simulink model "Simulink Library"  (R2018b)
settings: Solver=FixedStepAuto  StartTime=0.0  StopTime=10.0  RelTol=1e-3
undefined symbols (not defined in the file or in its folder): Battery, GYRO, LME, LRLI, MODE, MSE, PING, RME, RRLI
libraries: legoev3lib x36, simulink x33, dspstat3 x5, dspmtrx3 x3, fuzblock x2, simulink_extras x1
(part 2 of 2)

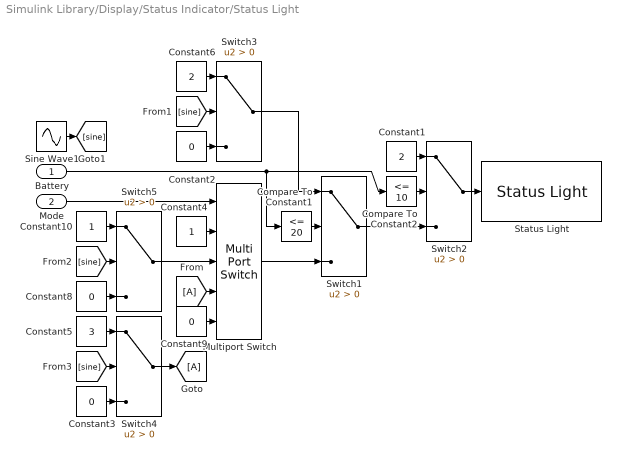
== system Simulink Library/Display/Status Indicator/Status Light ==
  Battery : Inport
  Mode : Inport  Port=2
  Compare To Constant1 : simulink/Logic and Bit Operations/Compare To Constant  relop=<=  const=20  OutDataTypeStr=boolean
  Compare To Constant2 : simulink/Logic and Bit Operations/Compare To Constant  relop=<=  const=10  OutDataTypeStr=boolean
  Constant1 : Constant  Value=2
  Constant10 : Constant
  Constant{2..3,8..9} (4 alike) : Constant  Value=0
  Constant4 : Constant
  Constant5 : Constant  Value=3
  Constant6 : Constant  Value=2
  Multiport Switch : MultiPortSwitch  DataPortOrder=Zero-based contiguous  Inputs=4  DiagnosticForDefault=None  zeroidx=on
  Sine Wave1 : Sin  SineType=Sample based  Samples=100  SampleTime=0.01
  Status Light : legoev3lib/Status Light
      settings: SourceProductName=Simulink Support Package for LEGO MINDSTORMS EV3 Hardware  SourceProductBaseCode=LEGOEV3
  Switch{1..5} (5 alike) : Switch  Criteria=u2 > Threshold
  wires:
  Multiport Switch/1 -> Switch1/3
  Compare To Constant2/1 -> Switch2/2
  Switch2/1 -> Status Light/1
  Battery/1 -> Compare To Constant2/1, Compare To Constant1/1
  Compare To Constant1/1 -> Switch1/2
  Switch1/1 -> Switch2/3
  Switch3/1 -> Switch1/1
  Mode/1 -> Multiport Switch/1
  Constant4/1 -> Multiport Switch/2
  Switch5/1 -> Multiport Switch/3
  [A] -> Multiport Switch/4
  Constant9/1 -> Multiport Switch/5
  [sine] -> Switch3/2
  Constant6/1 -> Switch3/1
  Constant2/1 -> Switch3/3
  Constant1/1 -> Switch2/1
  Constant5/1 -> Switch4/1
  [sine] -> Switch4/2
  Constant3/1 -> Switch4/3
  Constant10/1 -> Switch5/1
  [sine] -> Switch5/2
  Constant8/1 -> Switch5/3
  Switch4/1 -> [A]
  Sine Wave1/1 -> [sine]

== system Simulink Library/Motor Logic/Trim Logic/Trim High Spd ==
  Trim In : Inport
  Add2 : Sum  Inputs=+-
  Compare To Constant1 : simulink/Logic and Bit Operations/Compare To Constant  relop=>  const=0  OutDataTypeStr=boolean
  Compare To Constant2 : simulink/Logic and Bit Operations/Compare To Constant  relop=<  const=0  OutDataTypeStr=boolean
  Constant3 : Constant  Value=10
  Gain : Gain  Gain=-1
  Gain1 : Gain  Gain=-1
  Switch1 : Switch  Criteria=u2 > Threshold
  Switch2 : Switch  Criteria=u2 > Threshold
  Trim Right : Outport
  Trim Left : Outport  Port=2
  wires:
  Trim In/1 -> Add2/1
  Constant3/1 -> Add2/2
  Add2/1 -> Compare To Constant2/1, Switch2/1, Switch1/1, Compare To Constant1/1
  Compare To Constant1/1 -> Switch1/3, Switch1/2
  Compare To Constant2/1 -> Switch2/3, Switch2/2
  Switch1/1 -> Gain/1
  Gain/1 -> Trim Right/1
  Switch2/1 -> Gain1/1
  Gain1/1 -> Trim Left/1

== system Simulink Library/Motor Logic/Trim Logic/Trim Low Spd ==
  Trim In : Inport
  Add2 : Sum  Inputs=+-
  Compare To Constant1 : simulink/Logic and Bit Operations/Compare To Constant  relop=>  const=0  OutDataTypeStr=boolean
  Compare To Constant2 : simulink/Logic and Bit Operations/Compare To Constant  relop=<  const=0  OutDataTypeStr=boolean
  Constant3 : Constant  Value=10
  Switch1 : Switch  Criteria=u2 > Threshold
  Switch2 : Switch  Criteria=u2 > Threshold
  Trim Right : Outport
  Trim Left : Outport  Port=2
  wires:
  Trim In/1 -> Add2/1
  Constant3/1 -> Add2/2
  Add2/1 -> Compare To Constant2/1, Switch2/1, Switch1/1, Compare To Constant1/1
  Compare To Constant1/1 -> Switch1/3, Switch1/2
  Compare To Constant2/1 -> Switch2/3, Switch2/2
  Switch1/1 -> Trim Right/1
  Switch2/1 -> Trim Left/1

== system Simulink Library/PathTracking/Control Logic/Battery Bias ==
  Batt_Lvl : Inport
  Ceil : Rounding
  Constant : Constant
  Direct Lookup Table (n-D) : LookupNDDirect  NumberOfTableDimensions=1  Table=[0.256 0.128 0.064 0.032 0.016 0.008 0.004 0.002 0.001 0];
  Gain : Gain  Gain=0.1
  Sum : Sum  Inputs=|++
  Battery Bias : Outport
  wires:
  Direct Lookup Table (n-D)/1 -> Sum/1
  Constant/1 -> Sum/2
  Sum/1 -> Battery Bias/1
  Gain/1 -> Ceil/1
  Ceil/1 -> Direct Lookup Table (n-D)/1
  Batt_Lvl/1 -> Gain/1

== system Simulink Library/PathTracking/Control Logic/LP Filter && d//dt ==
  LightError : Inport
  Gain : Gain  Gain=1/0.01
  Low Pass Filter : DiscreteFilter  Numerator=[.2]  Denominator=[1 -0.8]
  Sum3 : Sum  Inputs=+-
  Unit Delay : UnitDelay  SampleTime=-1
  LightErrorDot : Outport
  wires:
  Unit Delay/1 -> Sum3/2
  Gain/1 -> Unit Delay/1, Sum3/1
  Sum3/1 -> LightErrorDot/1  "theta_dot"
  Low Pass Filter/1 -> Gain/1
  LightError/1 -> Low Pass Filter/1

== system Simulink Library/PathTracking/Control Logic/PID Bias ==
  RLI Error : Inport
  Abs : Abs
  Constant : Constant  Value=4
  Constant1 : Constant  Value=-4
  Switch1 : Switch  Criteria=u2 > Threshold  Threshold=30
  Switch2 : Switch  Criteria=u2 > Threshold
  PID_Bias : Outport
  wires:
  Switch1/1 -> PID_Bias/1
  RLI Error/1 -> Switch2/2, Abs/1
  Abs/1 -> Switch1/2
  Constant1/1 -> Switch2/1
  Constant/1 -> Switch2/3, Switch1/3
  Switch2/1 -> Switch1/1

== system Simulink Library/PathTracking/Control Logic/Real Time Speed Estimation ==
  LeftMotorEncoder : Inport
  RightMotorEncoder : Inport  Port=2
  Abs : Abs
  Add : Sum
  Degrees to Radians2 : simulink_extras/Transformations/Degrees to Radians
  Demux : Demux  Outputs=2
  Demux1 : Demux  Outputs=2
  Gain : Gain  Gain=0.5
  Low Pass Filter and derivative : Subsystem
  Low Pass Filter and derivative1 : Subsystem
  MinMax : MinMax  Function=max  Inputs=2
  Mux : Mux  Inputs=2
  Remove Initial Offset : Subsystem
  Vector Concatenate : Concatenate
  MotorSpeeds : Outport
  AvgSpeed : Outport  Port=2
  wires:
  Remove Initial Offset/1(x-x0) -> Demux/1
  LeftMotorEncoder/1 -> Mux/1
  RightMotorEncoder/1 -> Mux/2
  Demux/1 -> Low Pass Filter and derivative/1(theta)  "theta_L"
  Demux/2 -> Low Pass Filter and derivative1/1(theta)  "theta_R"
  Degrees to Radians2/1 -> Remove Initial Offset/1(x)
  Low Pass Filter and derivative1/1(theta_dot) -> Vector Concatenate/2, Add/2
  Gain/1 -> AvgSpeed/1
  Add/1 -> Gain/1
  Low Pass Filter and derivative/1(theta_dot) -> Vector Concatenate/1, Add/1
  Mux/1 -> Degrees to Radians2/1
  Vector Concatenate/1 -> Abs/1
  Abs/1 -> Demux1/1
  Demux1/1 -> MinMax/1
  Demux1/2 -> MinMax/2
  MinMax/1 -> MotorSpeeds/1

== system Simulink Library/PathTracking/Control Logic/Speed Bias ==
  Speed Reference : Inport
  Constant1 : Constant  Value=100
  Constant2 : Constant
  Divide : Product  Inputs=*/
  Switch : Switch  Criteria=u2 > Threshold  Threshold=55
  Linearized Gain : Outport
  wires:
  Constant2/1 -> Switch/3
  Speed Reference/1 -> Switch/2, Divide/1
  Divide/1 -> Switch/1
  Constant1/1 -> Divide/2
  Switch/1 -> Linearized Gain/1

== system Simulink Library/PathTracking/Control Logic/Real Time Speed Estimation/Low Pass Filter and derivative ==
  theta : Inport
  Gain : Gain  Gain=1/0.01
  Moving Average : dspstat3/Moving Average  Method=Sliding window  ForgettingFactorPort=off  SpecifyWindowLength=on  WindowLength=10  ForgettingFactor=0.9  SimulateUsing=Code generation
  Sum3 : Sum  Inputs=+-
  Unit Delay : UnitDelay  SampleTime=-1
  theta_dot : Outport
  wires:
  Unit Delay/1 -> Sum3/2
  Gain/1 -> Unit Delay/1, Sum3/1
  Sum3/1 -> theta_dot/1  "theta_dot"
  Moving Average/1 -> Gain/1
  theta/1 -> Moving Average/1

== system Simulink Library/PathTracking/Control Logic/Real Time Speed Estimation/Low Pass Filter and derivative1 ==
  theta : Inport
  Gain : Gain  Gain=1/0.01
  Moving Average : dspstat3/Moving Average  Method=Sliding window  ForgettingFactorPort=off  SpecifyWindowLength=on  WindowLength=10  ForgettingFactor=0.9  SimulateUsing=Code generation
  Sum3 : Sum  Inputs=+-
  Unit Delay : UnitDelay  SampleTime=-1
  theta_dot : Outport
  wires:
  Unit Delay/1 -> Sum3/2
  Gain/1 -> Unit Delay/1, Sum3/1
  Sum3/1 -> theta_dot/1  "theta_dot"
  Moving Average/1 -> Gain/1
  theta/1 -> Moving Average/1

== system Simulink Library/PathTracking/Control Logic/Real Time Speed Estimation/Remove Initial Offset ==
  x : Inport
  Constant : Constant  Value=0  OutDataTypeStr=boolean
  Store Offset : Subsystem  TreatAsAtomicUnit=on
  Sum2 : Sum  Inputs=-+|
  Unit Delay : UnitDelay  InitialCondition=1  SampleTime=-1
  x-x0 : Outport
  wires:
  Sum2/1 -> x-x0/1
  Unit Delay/1 -> Store Offset/Enable
  Constant/1 -> Unit Delay/1
  Store Offset/1(x0) -> Sum2/1
  x/1 -> Store Offset/1(x), Sum2/2

== system Simulink Library/PathTracking/Control Logic/Real Time Speed Estimation/Remove Initial Offset/Store Offset ==
  x : Inport
  Enable : EnablePort
  x0 : Outport  InitialOutput=0
  wires:
  x/1 -> x0/1
